simulink model "Square_HFI_Trigger"  (R2022b)
settings: Solver=FixedStepAuto  StartTime=0.0  StopTime=12  FixedStep=1e-7  RelTol=1e-3
undefined symbols (not defined in the file): DiscIntNeverNeededParam, sigbuilder_block
libraries: slpidlib x4, dspsigops x4, dsparch4 x2, simulink x2, spsDCVoltageSourceLib x1, spsPermanentMagnetSynchronousMachineLib x1, dspstat3 x1, spsUniversalBridgeLib x1, spspowerguiLib x1
settings Model: Creator=SSC  LastModifiedBy=SSC

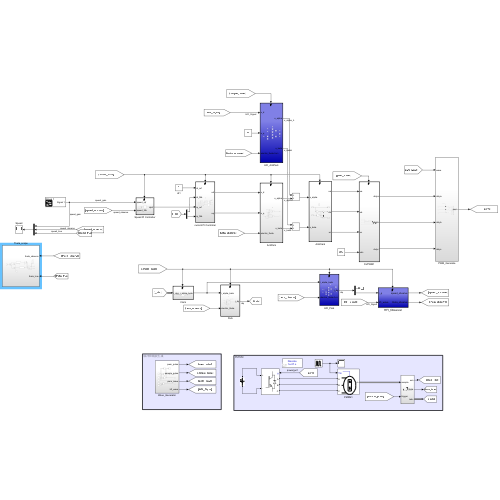
[thumbnail: Simulink's stored preview of the top-level diagram]
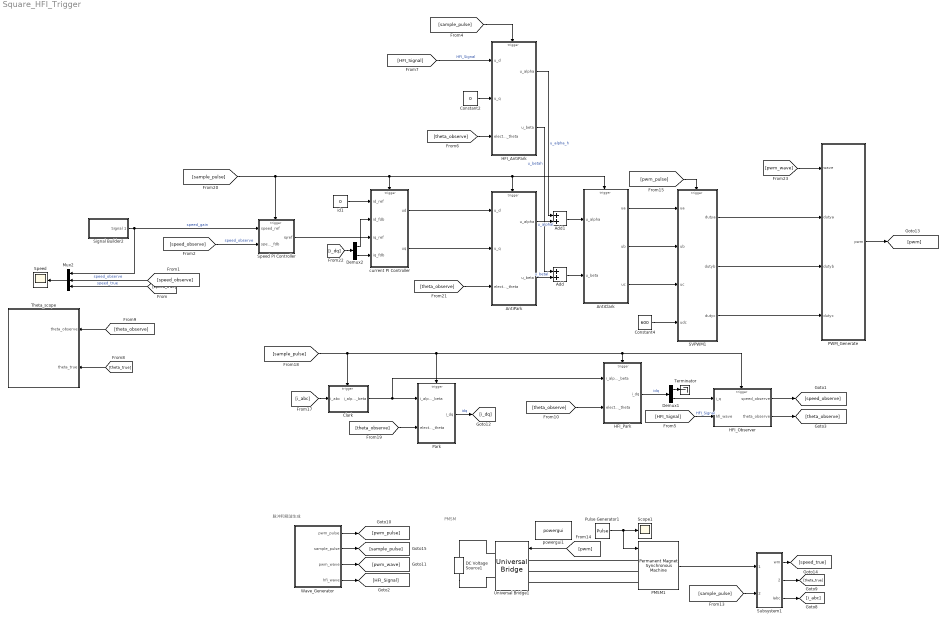
== system Square_HFI_Trigger ==
  note: 脉冲和载波生成
  note: PMSM
  Add : Sum
  Add1 : Sum
  AntiClark : Subsystem
  AntiPark : Subsystem
  Clark : Subsystem
  Constant2 : Constant  Value=0
  Constant4 : Constant  Value=600
  DC Voltage Source1 : spsDCVoltageSourceLib/DC Voltage Source  Amplitude=600  Measurements=None
  Demux1 : Demux  Outputs=2
  Demux2 : Demux  Outputs=2
  HFI_AntiPark : Subsystem
  HFI_Observer : Subsystem
  HFI_Park : Subsystem
  Mux2 : Mux  Inputs=3
  PMSM1 : spsPermanentMagnetSynchronousMachineLib/Permanent Magnet Synchronous Machine  NbPhases=3  FluxDistribution=Sinusoidal  RotorType=Salient-pole  MechanicalLoad=Torque Tm  PresetModel=No  ShowDetailedParameters=on  MeasurementBus=off  Resistance=0.91  Inductance=8.5e-3  dqInductances=[0.00396,0.00796]  La=8.5e-3  MachineConstant=Flux linkage established by magnets (V.s)  Flux=0.446  VoltageCst=161.7909  TorqueCst=1.338  Flat=120  Mechanical=[0.074 0.008 2 0]  PolePairs=4  InitialConditions=[0,0, 0,0]  InitialConditions5ph=[0 0 0 0 0 0]  RefAngle=Aligned with phase A axis (original Park)  IterativeDiscreteModel=Trapezoidal non iterative  TsBlock=-1  TsPowergui=0
  PWM_Generate : Subsystem
  Park : Subsystem
  Pulse Generator1 : DiscretePulseGenerator  PulseType=Time based  Period=3  PulseWidth=33.3  PhaseDelay=2.5
  SVPWM1 : Subsystem
  Scope1 : Scope
  Signal Builder2 : Subsystem  Tag=STV Subsys  LoadFcn=sigbuilder_block('load');  StartFcn=sigbuilder_block('start');  StopFcn=sigbuilder_block('stop');  ClipboardFcn=sigbuilder_block('clipboard');  mask(Sigbuilder block){tuvar=[0:10]}
      mask help: Simulink:masks:SigbuilderBlock_MD
      mask init:
      | if ~strcmp(get_param(bdroot(gcbh),'SimulationStatus'),'stopped') tuvar = sigbuilder_block('maskInit'); end
      settings: CopyFcn=sigbuilder_block('copy');  DeleteFcn=sigbuilder_block('delete');  ModelCloseFcn=sigbuilder_block('modelClose');  PreSaveFcn=sigbuilder_block('preSave');  PauseFcn=sigbuilder_block('pause');  ContinueFcn=sigbuilder_block('continue');  NameChangeFcn=sigbuilder_block('namechange');  OpenFcn=sigbuilder_block('open',[357 166.5 550.5 400.5 ]);  CloseFcn=sigbuilder_block('close');
      mask Display: plot(0, 0, 100, 100,[2, 2, 32, 32, 2], [68, 8, 8, 68, 68],[32, 2], [38, 38], [32, 19, 2],[53, 60, 44], [32, 17, 17, 2],[16, 16, 31, 31]);txt = getActiveGroup(gcbh);text(2, 100, txt,'verticalAlignment', 'top');
  Speed : Scope
  Speed PI Controller : Subsystem  TreatAsAtomicUnit=on
  Subsystem1 : Subsystem
  Terminator : Terminator
  Theta_scope : Subsystem
  Universal Bridge1 : spsUniversalBridgeLib/Universal Bridge  Arms=3  SnubberResistance=1e5  SnubberCapacitance=inf  Device=IGBT / Diodes  Ron=1e-3  Lon=0  ForwardVoltages="[  0  0  ]"  ForwardVoltage=0  GTOparameters=[ 10e-6 , 20e-6 ]  IGBTparameters=[ 1e-6 , 2e-6 ]  Measurements=None  Measurements_2=None  converterType=Rectifier
  Wave_Generator : Subsystem
  current PI Controller : Subsystem
  id1 : Constant  Value=0
  powergui1 : spspowerguiLib/powergui  Priority=1  SimulationMode=Discrete  SampleTime=1e-7  frequency=60  Iterations=50  frequencyindice=0  Pbase=100e6  ErrMax=1e-4  UnitsV=kV  UnitsW=MW  buscounter=0  FunctionMessages=off  echomessages=off  EnableUseOfTLC=off  CurrentSourceSwitches=off  DisableSnubberDevices=off  DisableRonSwitches=off  DisableVfSwitches=off  DisplayEquations=off  AutomaticDiscreteSolvers=off  SolverType=Tustin/Backward Euler (TBE)  Interpol=off  ExternalGateDelay=off  methode=off  Ts=100  x0status=blocks  SPID=on  SwTol=0  HookPort=off  NonlinearTolerance=1e-4  nMaxIteration=100  ContinueOnMaxIteration=off  RestoreLinks=warning  ResistiveCurrentMeasurement=off  Frange=[0:2:500]  Ylog=off  Xlog=on  ShowGrid=off  save=off  variable=ZData  structure=0  ZoomFFT=off  StartTime=0.0  cycles=1  DisplayStyle=1  fundamental=60  FreqAxis=off  MaxFrequency=1000  frequencyindicesteady=1  RmsSteady=1  display=off
  wires:
  Demux1/1 -> Terminator/1
  HFI_Observer/1(speed_observe) -> [speed_observe]
  HFI_Park/1(i_dq) -> Demux1/1  "idq"
  Constant2/1 -> HFI_AntiPark/2(u_q)
  [theta_observe] -> HFI_Park/2(electric_theta)
  [HFI_Signal] -> HFI_AntiPark/1(u_d)  "HFI_Signal"
  [theta_observe] -> HFI_AntiPark/3(electric_theta)
  Mux2/1 -> Speed/1
  [speed_true] -> Mux2/3  "speed_true"
  Demux1/2 -> HFI_Observer/1(i_q)
  [speed_observe] -> Mux2/2  "speed_observe"
  [i_abc] -> Clark/1(i_abc)
  [theta_observe] -> AntiPark/3(electric_theta)
  SVPWM1/3(dutyc) -> PWM_Generate/4(dutyc)
  [theta_observe] -> Park/2(electric_theta)
  current PI Controller/2(uq) -> AntiPark/2(u_q)
  Subsystem1/1(wm) -> [speed_true]
  Wave_Generator/3(pwm_wave) -> [pwm_wave]
  Wave_Generator/2(sample_pulse) -> [sample_pulse]
  [i_dq] -> Demux2/1
  [sample_pulse] -> Speed PI Controller/Trigger, AntiClark/Trigger, AntiPark/Trigger, current PI Controller/Trigger
  Demux2/2 -> current PI Controller/4(iq_fdb)
  Park/1(i_dq) -> [i_dq]  "idq"
  Subsystem1/2(theta) -> [theta_true]
  Speed PI Controller/1(iqref) -> current PI Controller/3(iq_ref)
  SVPWM1/2(dutyb) -> PWM_Generate/3(dutyb)
  Clark/1(i_alpha_beta) -> HFI_Park/1(i_alpha_beta), Park/1(i_alpha_beta)
  Pulse Generator1/1 -> PMSM1/1, Scope1/1
  AntiClark/2(ub) -> SVPWM1/2(ub)
  Signal Builder2/1(Signal 1) -> Mux2/1, Speed PI Controller/1(speed_ref)  "speed_gain"
  PMSM1/1 -> Subsystem1/1(sample)
  Constant4/1 -> SVPWM1/4(udc)
  [pwm_wave] -> PWM_Generate/1(wave)
  [pwm] -> Universal Bridge1/1
  [pwm_pulse] -> SVPWM1/Trigger
  current PI Controller/1(ud) -> AntiPark/1(u_d)
  id1/1 -> current PI Controller/1(id_ref)
  Subsystem1/3(Iabc) -> [i_abc]
  Demux2/1 -> current PI Controller/2(id_fdb)
  PWM_Generate/1(pwm) -> [pwm]
  Wave_Generator/1(pwm_pulse) -> [pwm_pulse]
  [sample_pulse] -> Subsystem1/2(trigger)
  AntiClark/3(uc) -> SVPWM1/3(uc)
  [sample_pulse] -> HFI_Observer/Trigger, HFI_Park/Trigger, Park/Trigger, Clark/Trigger
  SVPWM1/1(dutya) -> PWM_Generate/2(dutya)
  AntiPark/1(u_alpha) -> Add1/2  "u_alphal"
  AntiPark/2(u_beta) -> Add/2  "u_betal"
  Add1/1 -> AntiClark/1(u_alpha)
  AntiClark/1(ua) -> SVPWM1/1(ua)
  Add/1 -> AntiClark/2(u_beta)
  [sample_pulse] -> HFI_AntiPark/Trigger
  Wave_Generator/4(hfi_wave) -> [HFI_Signal]
  [HFI_Signal] -> HFI_Observer/2(hfi_wave)  "HFI_Signal"
  HFI_Observer/2(theta_observe) -> [theta_observe]
  HFI_AntiPark/2(u_beta) -> Add/1  "u_betah"
  HFI_AntiPark/1(u_alpha) -> Add1/1  "u_alpha_h"
  [speed_observe] -> Speed PI Controller/2(speed_fdb)  "speed_observe"
  [theta_observe] -> Theta_scope/1(theta_observe)
  [theta_true] -> Theta_scope/2(theta_true)
  connections:
  PMSM1/LConn1 -- Universal Bridge1/LConn1
  PMSM1/LConn2 -- Universal Bridge1/LConn2
  Universal Bridge1/RConn1 -- DC Voltage Source1/RConn1
  PMSM1/LConn3 -- Universal Bridge1/LConn3
  DC Voltage Source1/LConn1 -- Universal Bridge1/RConn2

== system Square_HFI_Trigger/AntiClark ==
  u_alpha : Inport
  u_beta : Inport  Port=2
  Trigger : TriggerPort  VariantControl=(inherit)
  Gain : Gain  Gain=-1/2
  Gain1 : Gain  Gain=sqrt(3)/2
  Sum : Sum  Inputs=|++
  Sum1 : Sum  Inputs=-+|
  ua : Outport
  ub : Outport  Port=2
  uc : Outport  Port=3
  wires:
  Sum1/1 -> uc/1
  Gain1/1 -> Sum1/1, Sum/2
  Sum/1 -> ub/1
  Gain/1 -> Sum/1, Sum1/2
  u_beta/1 -> Gain1/1
  u_alpha/1 -> ua/1, Gain/1

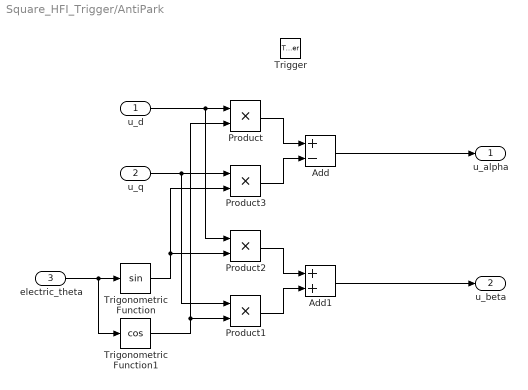
== system Square_HFI_Trigger/AntiPark ==
  u_d : Inport
  u_q : Inport  Port=2
  electric_theta : Inport  Port=3
  Trigger : TriggerPort  VariantControl=(inherit)
  Add : Sum  Inputs=+-
  Add1 : Sum
  Product{,1..3} (4 alike) : Product
  Trigonometric Function : Trigonometry
  Trigonometric Function1 : Trigonometry  Operator=cos
  u_alpha : Outport
  u_beta : Outport  Port=2
  wires:
  electric_theta/1 -> Trigonometric Function1/1, Trigonometric Function/1
  u_d/1 -> Product2/1, Product/1
  Trigonometric Function1/1 -> Product/2, Product1/2
  u_q/1 -> Product1/1, Product3/1
  Trigonometric Function/1 -> Product2/2, Product3/2
  Product/1 -> Add/1
  Product3/1 -> Add/2
  Add/1 -> u_alpha/1
  Product2/1 -> Add1/1
  Product1/1 -> Add1/2
  Add1/1 -> u_beta/1

== system Square_HFI_Trigger/Clark ==
  i_abc : Inport
  Trigger : TriggerPort  VariantControl=(inherit)
  Clark : Subsystem
  Demux : Demux  Outputs=3
  Mux6 : Mux  Inputs=2
  i_alpha_beta : Outport  VectorParamsAs1DForOutWhenUnconnected=off
  wires:
  Clark/2(I_beta) -> Mux6/2
  Mux6/1 -> i_alpha_beta/1
  Demux/3 -> Clark/3(I_c)
  Clark/1(I_alpha) -> Mux6/1
  i_abc/1 -> Demux/1
  Demux/2 -> Clark/2(I_b)
  Demux/1 -> Clark/1(I_a)

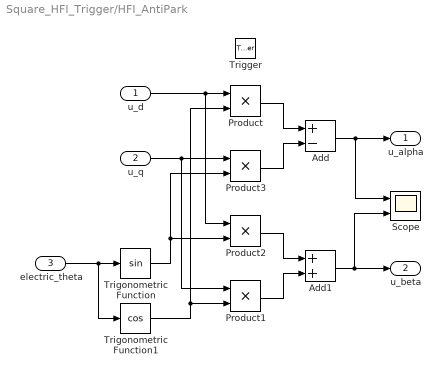
== system Square_HFI_Trigger/HFI_AntiPark ==
  u_d : Inport
  u_q : Inport  Port=2
  electric_theta : Inport  Port=3  LatchByDelayingOutsideSignal=on
  Trigger : TriggerPort  VariantControl=(inherit)
  Add : Sum  Inputs=+-
  Add1 : Sum
  Product{,1..3} (4 alike) : Product
  Scope : Scope  NumInputPorts=2
  Trigonometric Function : Trigonometry
  Trigonometric Function1 : Trigonometry  Operator=cos
  u_alpha : Outport
  u_beta : Outport  Port=2
  wires:
  electric_theta/1 -> Trigonometric Function1/1, Trigonometric Function/1
  u_d/1 -> Product2/1, Product/1
  Trigonometric Function1/1 -> Product/2, Product1/2
  u_q/1 -> Product1/1, Product3/1
  Trigonometric Function/1 -> Product2/2, Product3/2
  Product/1 -> Add/1
  Product3/1 -> Add/2
  Add/1 -> Scope/1, u_alpha/1
  Product2/1 -> Add1/1
  Product1/1 -> Add1/2
  Add1/1 -> Scope/2, u_beta/1

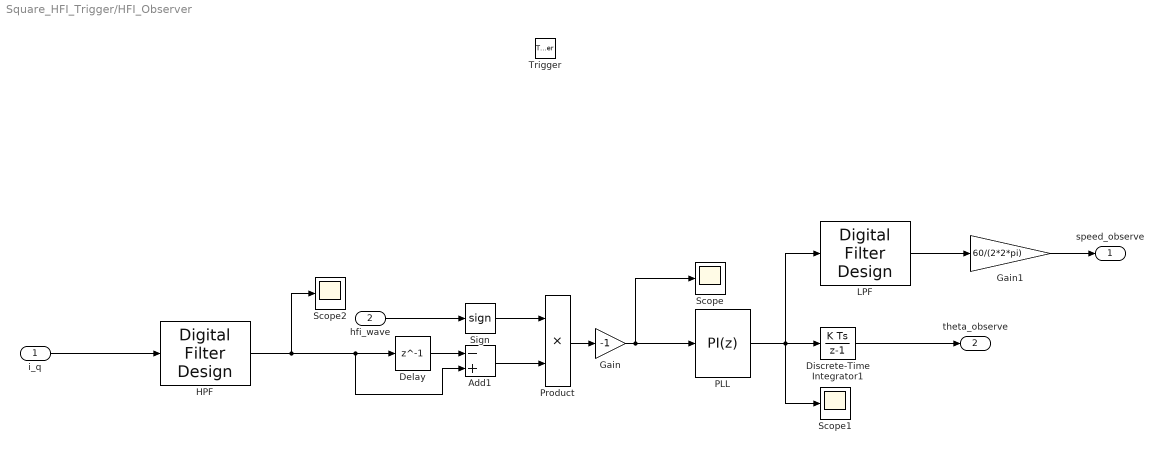
== system Square_HFI_Trigger/HFI_Observer ==
  i_q : Inport
  hfi_wave : Inport  Port=2
  Trigger : TriggerPort  VariantControl=(inherit)
  Add1 : Sum  Inputs=-+
  Delay : Delay  DelayLength=1  InitialCondition=0
  Discrete-Time Integrator1 : DiscreteIntegrator  SampleTime=-1  ICPrevOutput=DiscIntNeverNeededParam  ICPrevScaledInput=DiscIntNeverNeededParam
  Gain : Gain  Gain=-1
  Gain1 : Gain  Gain=60/(2*2*pi)
  HPF : dsparch4/Digital Filter Design  mwdsp_browser_bugfix_var=off
  LPF : dsparch4/Digital Filter Design  mwdsp_browser_bugfix_var=off
  PLL : slpidlib/PID Controller  Controller=PI  Form=Parallel  TimeDomain=Discrete-time  UseExternalTs=off  SampleTime=-1  IntegratorMethod=Forward Euler  FilterMethod=Forward Euler  ControllerParametersSource=internal  P=10000  I=16000/2  UseKiTs=off  D=0  N=100  UseFilter=on  TunerSelectOption=Transfer Function Based (PID Tuner App)  InitialConditionSource=internal  InitialConditionForIntegrator=0  InitialConditionForFilter=0  DifferentiatorICPrevScaledInput=0  ExternalReset=none  TrackingMode=off  Kt=1  LimitOutput=off  SatLimitsSource=internal  UpperSaturationLimit=100*2*pi  LowerSaturationLimit=-100*2*pi  LinearizeAsGain=on  AntiWindupMode=clamping  Kb=1  LimitIntegrator=off  UpperIntegratorSaturationLimit=inf  LowerIntegratorSaturationLimit=-inf  POutMin=[]  POutMax=[]  IOutMin=[]  IOutMax=[]  DOutMin=[]  DOutMax=[]  NOutMin=[]  NOutMax=[]  SumOutMin=[]  SumOutMax=[]  SaturationOutMin=[]  SaturationOutMax=[]  PParamMin=[]  PParamMax=[]  IParamMin=[]  IParamMax=[]  DParamMin=[]  DParamMax=[]  NParamMin=[]  NParamMax=[]  KbParamMin=[]  KbParamMax=[]  KtParamMin=[]  KtParamMax=[]  KbOutMin=[]  KbOutMax=[]  KtOutMin=[]  KtOutMax=[]  IntegratorOutMin=[]  IntegratorOutMax=[]  FilterOutMin=[]  FilterOutMax=[]  SumI1OutMin=[]  SumI1OutMax=[]  SumI2OutMin=[]  SumI2OutMax=[]  SumI3OutMin=[]  SumI3OutMax=[]  SumI4OutMin=[]  SumI4OutMax=[]  SumDOutMin=[]  SumDOutMax=[]  DifferentiatorOutMin=[]  DifferentiatorOutMax=[]  FilterDiffOutCoefMin=[]  FilterDiffOutCoefMax=[]  ReciprocalOutMin=[]  ReciprocalOutMax=[]  SumDenOutMin=[]  SumDenOutMax=[]  SumNumOutMin=[]  SumNumOutMax=[]  DivideOutMin=[]  DivideOutMax=[]  UdiffTsProdOutMin=[]  UdiffTsProdOutMax=[]  NTsProdOutMin=[]  NTsProdOutMax=[]  UintegralTsProdOutMin=[]  UintegralTsProdOutMax=[]  UngainTsProdOutMin=[]  UngainTsProdOutMax=[]  ClampingZeroOutDataTypeStr=Inherit: Inherit via back propagation  ClampingZeroOutMin=[]  ClampingZeroOutMax=[]  FilterDenConstantOutDataTypeStr=Inherit: Inherit via back propagation  FilterDenConstantOutMin=[]  FilterDenConstantOutMax=[]  PCopyOutDataTypeStr=Inherit: Inherit via back propagation  PCopyOutMin=[]  PCopyOutMax=[]  NCopyOutDataTypeStr=Inherit: Inherit via back propagation  NCopyOutMin=[]  NCopyOutMax=[]  IntegratorContinuousStateAttributes=''  IntegratorStateMustResolveToSignalObject=off  IntegratorRTWStateStorageClass=Auto  FilterContinuousStateAttributes=''  FilterStateMustResolveToSignalObject=off  FilterRTWStateStorageClass=Auto  ParallelPVariant=InternalParameters  IdealPVariant=Disabled  IVariant=InternalParameters  DVariant=Disabled  IntegratorVariant=Discrete  SatVariant=Disabled  AWVariant=Passthrough  PCopyVariant=Disabled  TRVariant=Disabled  FdbkBlocksVariant=Forward  IdealPFdbkVariant=Disabled  SatFdbkVariant=Disabled  DerivativeFilterVariant=Disabled  NVariant=Disabled  NCopyVariant=Disabled_SignalSpec  FilterICVariant=Disabled  IntegratorICVariant=InternalICs  ExternalResetVariant=Disabled  TRSumVariant=Passthrough  SumFdbkVariant=Disabled  SumVariant=Sum_PI  TsampFilterVariant=InternalTs  TsampNgainVariant=Passthrough  TsampIntegralVariant=Passthrough  ExternalSaturationOutDataTypeStr=Inherit: Same as second input
  Product : Product
  Scope : Scope
  Scope1 : Scope
  Scope2 : Scope
  Sign : Signum
  speed_observe : Outport  VectorParamsAs1DForOutWhenUnconnected=off
  theta_observe : Outport  Port=2  VectorParamsAs1DForOutWhenUnconnected=off
  wires:
  PLL/1 -> Discrete-Time Integrator1/1, Scope1/1, LPF/1
  Gain1/1 -> speed_observe/1
  LPF/1 -> Gain1/1
  Delay/1 -> Add1/1
  Add1/1 -> Product/2
  Sign/1 -> Product/1
  Product/1 -> Gain/1
  i_q/1 -> HPF/1
  HPF/1 -> Scope2/1, Add1/2, Delay/1
  hfi_wave/1 -> Sign/1
  Discrete-Time Integrator1/1 -> theta_observe/1
  Gain/1 -> Scope/1, PLL/1

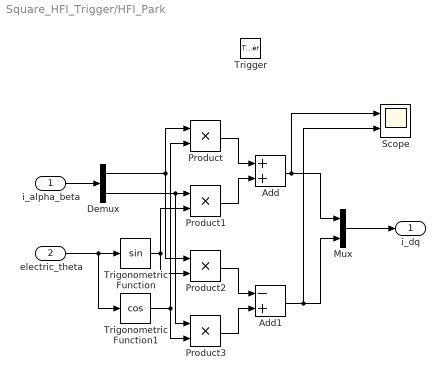
== system Square_HFI_Trigger/HFI_Park ==
  i_alpha_beta : Inport
  electric_theta : Inport  Port=2  LatchByDelayingOutsideSignal=on
  Trigger : TriggerPort  VariantControl=(inherit)
  Add : Sum
  Add1 : Sum  Inputs=-+
  Demux : Demux  Outputs=2
  Mux : Mux  Inputs=2
  Product{,1..3} (4 alike) : Product
  Scope : Scope  NumInputPorts=2
  Trigonometric Function : Trigonometry
  Trigonometric Function1 : Trigonometry  Operator=cos
  i_dq : Outport
  wires:
  electric_theta/1 -> Trigonometric Function1/1, Trigonometric Function/1
  Trigonometric Function1/1 -> Product3/2, Product/2
  Demux/2 -> Product3/1, Product1/1
  Trigonometric Function/1 -> Product2/2, Product1/2
  Product/1 -> Add/1
  Product1/1 -> Add/2
  Product2/1 -> Add1/1
  Product3/1 -> Add1/2
  Add/1 -> Scope/1, Mux/1
  Add1/1 -> Scope/2, Mux/2
  Demux/1 -> Product/1, Product2/1
  i_alpha_beta/1 -> Demux/1
  Mux/1 -> i_dq/1

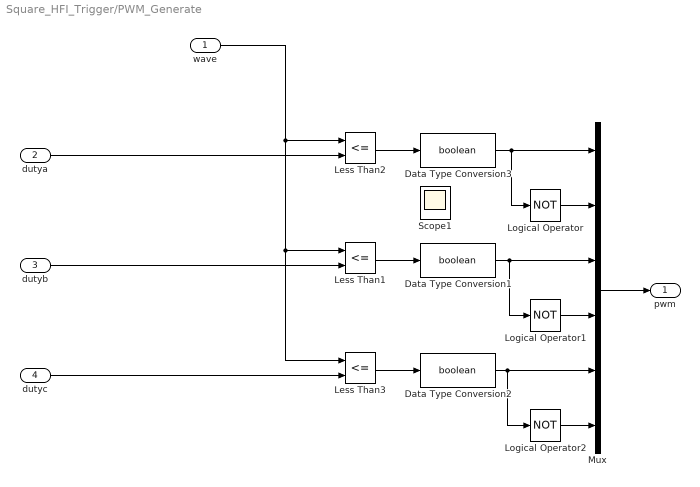
== system Square_HFI_Trigger/PWM_Generate ==
  wave : Inport
  dutya : Inport  Port=2
  dutyb : Inport  Port=3
  dutyc : Inport  Port=4
  Data Type Conversion1 : DataTypeConversion  OutDataTypeStr=boolean  SaturateOnIntegerOverflow=off  RndMeth=Floor
  Data Type Conversion2 : DataTypeConversion  OutDataTypeStr=boolean  SaturateOnIntegerOverflow=off  RndMeth=Floor
  Data Type Conversion3 : DataTypeConversion  OutDataTypeStr=boolean  SaturateOnIntegerOverflow=off  RndMeth=Floor
  Less Than1 : RelationalOperator  Operator=<=  OutDataTypeStr=boolean  RndMeth=Simplest  InputSameDT=off
  Less Than2 : RelationalOperator  Operator=<=  OutDataTypeStr=boolean  RndMeth=Simplest  InputSameDT=off
  Less Than3 : RelationalOperator  Operator=<=  OutDataTypeStr=boolean  RndMeth=Simplest  InputSameDT=off
  Logical Operator : Logic  Operator=NOT  AllPortsSameDT=off  OutDataTypeStr=boolean
  Logical Operator1 : Logic  Operator=NOT  AllPortsSameDT=off  OutDataTypeStr=boolean
  Logical Operator2 : Logic  Operator=NOT  AllPortsSameDT=off  OutDataTypeStr=boolean
  Mux : Mux  Inputs=6
  Scope1 : Scope  NumInputPorts=2
  pwm : Outport
  wires:
  wave/1 -> Less Than3/1, Less Than1/1, Less Than2/1
  Less Than1/1 -> Data Type Conversion1/1
  Less Than2/1 -> Data Type Conversion3/1
  dutyb/1 -> Less Than1/2
  Less Than3/1 -> Data Type Conversion2/1
  dutya/1 -> Less Than2/2
  dutyc/1 -> Less Than3/2
  Data Type Conversion3/1 -> Logical Operator/1, Mux/1
  Logical Operator/1 -> Mux/2
  Data Type Conversion1/1 -> Logical Operator1/1, Mux/3
  Data Type Conversion2/1 -> Logical Operator2/1, Mux/5
  Logical Operator2/1 -> Mux/6
  Mux/1 -> pwm/1
  Logical Operator1/1 -> Mux/4

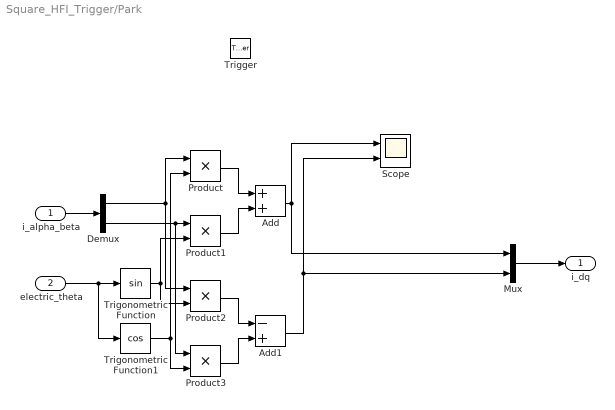
== system Square_HFI_Trigger/Park ==
  i_alpha_beta : Inport
  electric_theta : Inport  Port=2
  Trigger : TriggerPort  VariantControl=(inherit)
  Add : Sum
  Add1 : Sum  Inputs=-+
  Demux : Demux  Outputs=2
  Mux : Mux  Inputs=2
  Product{,1..3} (4 alike) : Product
  Scope : Scope  NumInputPorts=2
  Trigonometric Function : Trigonometry
  Trigonometric Function1 : Trigonometry  Operator=cos
  i_dq : Outport
  wires:
  electric_theta/1 -> Trigonometric Function1/1, Trigonometric Function/1
  Trigonometric Function1/1 -> Product3/2, Product/2
  Demux/2 -> Product3/1, Product1/1
  Trigonometric Function/1 -> Product2/2, Product1/2
  Product/1 -> Add/1
  Product1/1 -> Add/2
  Product2/1 -> Add1/1
  Product3/1 -> Add1/2
  Demux/1 -> Product/1, Product2/1
  i_alpha_beta/1 -> Demux/1
  Mux/1 -> i_dq/1
  Add/1 -> Mux/1, Scope/1
  Add1/1 -> Mux/2, Scope/2

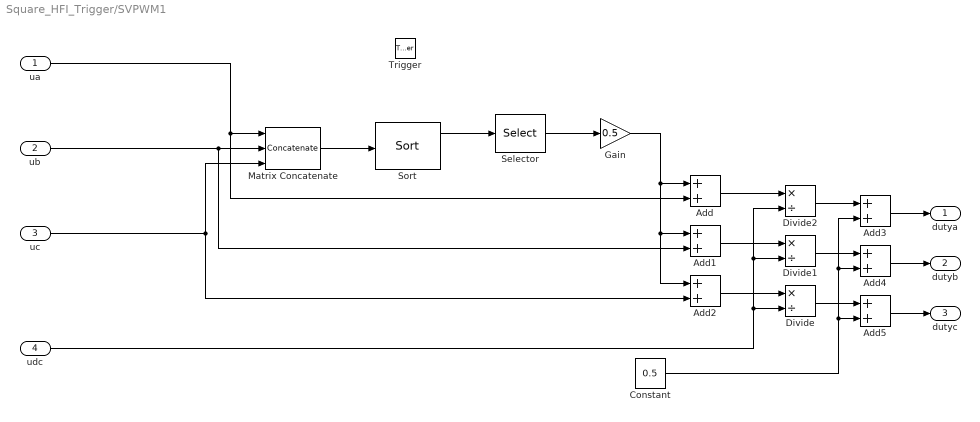
== system Square_HFI_Trigger/SVPWM1 ==
  ua : Inport
  ub : Inport  Port=2
  uc : Inport  Port=3
  udc : Inport  Port=4
  Trigger : TriggerPort  VariantControl=(inherit)
  Add{,1..5} (6 alike) : Sum
  Constant : Constant  Value=0.5
  Divide : Product  Inputs=*/
  Divide1 : Product  Inputs=*/
  Divide2 : Product  Inputs=*/
  Gain : Gain  Gain=0.5
  Matrix Concatenate : Concatenate  NumInputs=3  ConcatenateDimension=2
  Selector : Selector  InputPortWidth=3  IndexOptions=Index vector (dialog)  Indices=2  OutputSizes=1
  Sort : dspstat3/Sort  otype=Value and Index  dir=Ascending  sortAlg=Quick sort  roundingMode=Floor  overflowMode=off  accumDataTypeStr=Inherit: Same as product output  accumLastDataTypeStr=Inherit: Same as product output
  dutya : Outport
  dutyb : Outport  Port=2
  dutyc : Outport  Port=3
  wires:
  Selector/1 -> Gain/1
  udc/1 -> Divide/2, Divide2/2, Divide1/2
  Add1/1 -> Divide1/1
  Sort/1 -> Selector/1
  Matrix Concatenate/1 -> Sort/1
  Add2/1 -> Divide/1
  Gain/1 -> Add2/1, Add1/1, Add/1
  ua/1 -> Add/2, Matrix Concatenate/1
  Add/1 -> Divide2/1
  uc/1 -> Matrix Concatenate/3, Add2/2
  ub/1 -> Add1/2, Matrix Concatenate/2
  Divide2/1 -> Add3/1
  Divide1/1 -> Add4/1
  Divide/1 -> Add5/1
  Constant/1 -> Add5/2, Add4/2, Add3/2
  Add3/1 -> dutya/1
  Add4/1 -> dutyb/1
  Add5/1 -> dutyc/1

== system Square_HFI_Trigger/Signal Builder2 ==
  Demux : Demux  Tag=STV Demux  Outputs=1
      settings: DisplayOption=none
  FromWs : FromWorkspace  Tag=STV FromWs  VariableName=tuvar
      SigBuilderData=|
      | common.afterFinalStr = 'Extrapolate'
      | common.sampleTime = 0
      | dataSet.timeRange = [0 13]
      | dataSet.name = 'Group 1'
      | sbobj.Groups.Name = 'Group 1'
      | sbobj.Groups.Signals.Name = 'Signal 1'
      | sbobj.Groups.Signals.XData = [0 0.5 0.51 8 8 13]
      | sbobj.Groups.Signals.YData = [0 0 50 50 40 40]
      | sbobj.Groups.TimeRange = [0 13]
  Signal 1 : Outport  Tag=STV Outport
  wires:
  FromWs/1 -> Demux/1
  Demux/1 -> Signal 1/1

== system Square_HFI_Trigger/Speed PI Controller ==
  speed_ref : Inport
  speed_fdb : Inport  Port=2
  Trigger : TriggerPort  VariantControl=(inherit)
  Speed PI Controller : slpidlib/PID Controller  Controller=PI  Form=Parallel  TimeDomain=Discrete-time  UseExternalTs=off  SampleTime=-1  IntegratorMethod=Forward Euler  FilterMethod=Forward Euler  ControllerParametersSource=internal  P=3.786/30  I=44.84/30/2  UseKiTs=off  D=0  N=100  UseFilter=on  TunerSelectOption=Transfer Function Based (PID Tuner App)  InitialConditionSource=internal  InitialConditionForIntegrator=0  InitialConditionForFilter=0  DifferentiatorICPrevScaledInput=0  ExternalReset=none  TrackingMode=off  Kt=1  LimitOutput=off  SatLimitsSource=internal  UpperSaturationLimit=5.65  LowerSaturationLimit=-5.65  LinearizeAsGain=on  AntiWindupMode=clamping  Kb=1  LimitIntegrator=off  UpperIntegratorSaturationLimit=inf  LowerIntegratorSaturationLimit=-inf  POutMin=[]  POutMax=[]  IOutMin=[]  IOutMax=[]  DOutMin=[]  DOutMax=[]  NOutMin=[]  NOutMax=[]  SumOutMin=[]  SumOutMax=[]  SaturationOutMin=[]  SaturationOutMax=[]  PParamMin=[]  PParamMax=[]  IParamMin=[]  IParamMax=[]  DParamMin=[]  DParamMax=[]  NParamMin=[]  NParamMax=[]  KbParamMin=[]  KbParamMax=[]  KtParamMin=[]  KtParamMax=[]  KbOutMin=[]  KbOutMax=[]  KtOutMin=[]  KtOutMax=[]  IntegratorOutMin=[]  IntegratorOutMax=[]  FilterOutMin=[]  FilterOutMax=[]  SumI1OutMin=[]  SumI1OutMax=[]  SumI2OutMin=[]  SumI2OutMax=[]  SumI3OutMin=[]  SumI3OutMax=[]  SumI4OutMin=[]  SumI4OutMax=[]  SumDOutMin=[]  SumDOutMax=[]  DifferentiatorOutMin=[]  DifferentiatorOutMax=[]  FilterDiffOutCoefMin=[]  FilterDiffOutCoefMax=[]  ReciprocalOutMin=[]  ReciprocalOutMax=[]  SumDenOutMin=[]  SumDenOutMax=[]  SumNumOutMin=[]  SumNumOutMax=[]  DivideOutMin=[]  DivideOutMax=[]  UdiffTsProdOutMin=[]  UdiffTsProdOutMax=[]  NTsProdOutMin=[]  NTsProdOutMax=[]  UintegralTsProdOutMin=[]  UintegralTsProdOutMax=[]  UngainTsProdOutMin=[]  UngainTsProdOutMax=[]  ClampingZeroOutDataTypeStr=Inherit: Inherit via back propagation  ClampingZeroOutMin=[]  ClampingZeroOutMax=[]  FilterDenConstantOutDataTypeStr=Inherit: Inherit via back propagation  FilterDenConstantOutMin=[]  FilterDenConstantOutMax=[]  PCopyOutDataTypeStr=Inherit: Inherit via back propagation  PCopyOutMin=[]  PCopyOutMax=[]  NCopyOutDataTypeStr=Inherit: Inherit via back propagation  NCopyOutMin=[]  NCopyOutMax=[]  IntegratorContinuousStateAttributes=''  IntegratorStateMustResolveToSignalObject=off  IntegratorRTWStateStorageClass=Auto  FilterContinuousStateAttributes=''  FilterStateMustResolveToSignalObject=off  FilterRTWStateStorageClass=Auto  ParallelPVariant=InternalParameters  IdealPVariant=Disabled  IVariant=InternalParameters  DVariant=Disabled  IntegratorVariant=Discrete  SatVariant=Disabled  AWVariant=Passthrough  PCopyVariant=Disabled  TRVariant=Disabled  FdbkBlocksVariant=Forward  IdealPFdbkVariant=Disabled  SatFdbkVariant=Disabled  DerivativeFilterVariant=Disabled  NVariant=Disabled  NCopyVariant=Disabled_SignalSpec  FilterICVariant=Disabled  IntegratorICVariant=InternalICs  ExternalResetVariant=Disabled  TRSumVariant=Passthrough  SumFdbkVariant=Disabled  SumVariant=Sum_PI  TsampFilterVariant=InternalTs  TsampNgainVariant=Passthrough  TsampIntegralVariant=Passthrough  ExternalSaturationOutDataTypeStr=Inherit: Same as second input
  Sum3 : Sum  Inputs=|+-
  iqref : Outport
  wires:
  Sum3/1 -> Speed PI Controller/1
  Speed PI Controller/1 -> iqref/1
  speed_ref/1 -> Sum3/1
  speed_fdb/1 -> Sum3/2

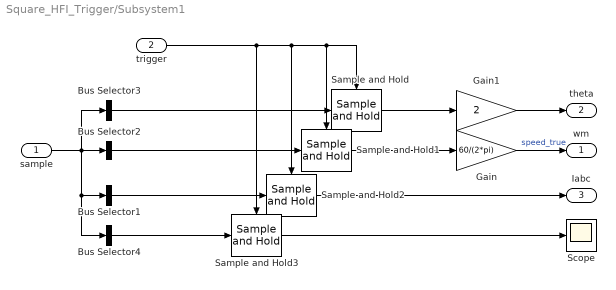
== system Square_HFI_Trigger/Subsystem1 ==
  sample : Inport
  trigger : Inport  Port=2
  Bus Selector1 : BusSelector  OutputSignals=Stator current is_a (A),Stator current is_b (A),Stator current is_c (A)  OutputAsBus=on
  Bus Selector2 : BusSelector  OutputSignals=Rotor speed wm (rad/s)  OutputAsBus=on
  Bus Selector3 : BusSelector  OutputSignals=Rotor angle thetam (rad)  OutputAsBus=on
  Bus Selector4 : BusSelector  OutputSignals=Rotor speed wm (rad/s)  OutputAsBus=on
  Gain : Gain  Gain=60/(2*pi)
  Gain1 : Gain  Gain=2
  Sample and Hold{,1..3} (4 alike) : dspsigops/Sample and Hold  trig=Rising edge  initCond=0  latchinput=off
  Scope : Scope
  wm : Outport  VectorParamsAs1DForOutWhenUnconnected=off
  theta : Outport  Port=2  VectorParamsAs1DForOutWhenUnconnected=off
  Iabc : Outport  Port=3  VectorParamsAs1DForOutWhenUnconnected=off
  wires:
  sample/1 -> Bus Selector4/1, Bus Selector1/1, Bus Selector3/1, Bus Selector2/1
  Gain/1 -> wm/1  "speed_true"
  Gain1/1 -> theta/1
  Sample and Hold/1 -> Gain1/1
  Bus Selector3/1 -> Sample and Hold/1
  Sample and Hold1/1 -> Gain/1
  Bus Selector2/1 -> Sample and Hold1/1
  Bus Selector1/1 -> Sample and Hold2/1
  Sample and Hold2/1 -> Iabc/1
  Bus Selector4/1 -> Sample and Hold3/1
  Sample and Hold3/1 -> Scope/1
  trigger/1 -> Sample and Hold3/Trigger, Sample and Hold2/Trigger, Sample and Hold1/Trigger, Sample and Hold/Trigger

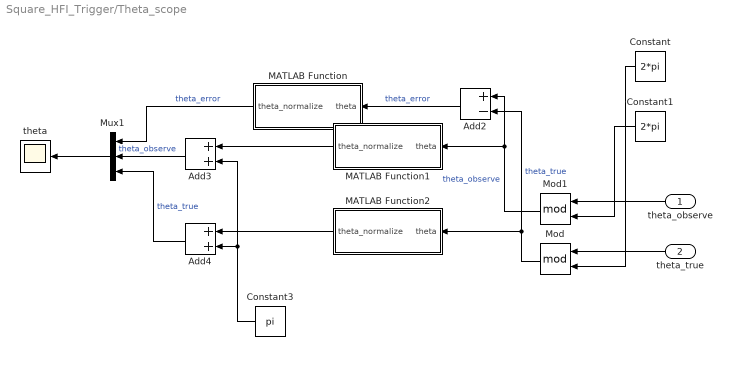
== system Square_HFI_Trigger/Theta_scope ==
  theta_observe : Inport
  theta_true : Inport  Port=2
  Add2 : Sum  Inputs=+-
  Add3 : Sum
  Add4 : Sum
  Constant : Constant  Value=2*pi
  Constant1 : Constant  Value=2*pi
  Constant3 : Constant  Value=pi
  MATLAB Function : MATLAB Function  TreatAsAtomicUnit=on
  MATLAB Function1 : MATLAB Function  TreatAsAtomicUnit=on
  MATLAB Function2 : MATLAB Function  TreatAsAtomicUnit=on
  Mod : Math  Operator=mod  SignedPower=on
  Mod1 : Math  Operator=mod  SignedPower=on
  Mux1 : Mux  Inputs=3
  theta : Scope
  wires:
  Add4/1 -> Mux1/3  "theta_true"
  Constant1/1 -> Mod1/2
  Constant/1 -> Mod/2
  MATLAB Function2/1(theta_normalize) -> Add4/1
  Mod/1 -> Add2/2, MATLAB Function2/1(theta)  "theta_true"
  Mux1/1 -> theta/1
  theta_observe/1 -> Mod1/1
  Constant3/1 -> Add4/2, Add3/2
  MATLAB Function/1(theta_normalize) -> Mux1/1  "theta_error"
  MATLAB Function1/1(theta_normalize) -> Add3/1
  Mod1/1 -> Add2/1, MATLAB Function1/1(theta)  "theta_observe"
  Add3/1 -> Mux1/2  "theta_observe"
  Add2/1 -> MATLAB Function/1(theta)  "theta_error"
  theta_true/1 -> Mod/1

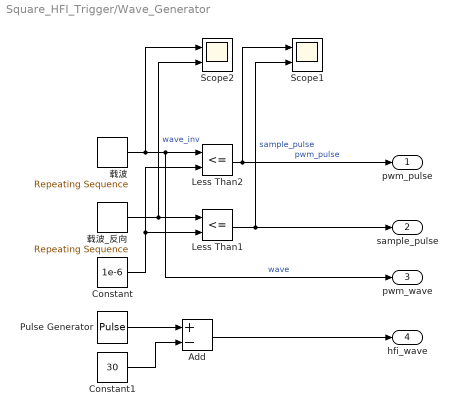
== system Square_HFI_Trigger/Wave_Generator ==
  Add : Sum  Inputs=+-
  Constant : Constant  Value=1e-6
  Constant1 : Constant  Value=30
  Less Than1 : RelationalOperator  Operator=<=  OutDataTypeStr=boolean  RndMeth=Simplest  InputSameDT=off
  Less Than2 : RelationalOperator  Operator=<=  OutDataTypeStr=boolean  RndMeth=Simplest  InputSameDT=off
  Pulse Generator : DiscretePulseGenerator  PulseType=Time based  Amplitude=60  Period=2e-4  PulseWidth=50
  Scope1 : Scope  NumInputPorts=2
  Scope2 : Scope  NumInputPorts=2
  载波 : simulink/Sources/Repeating Sequence  rep_seq_t=[0 0.5e-4 1e-4]  rep_seq_y=[0 1 0]
  载波_反向 : simulink/Sources/Repeating Sequence  rep_seq_t=[0 0.5e-4 1e-4]  rep_seq_y=[1 0 1]
  pwm_pulse : Outport
  sample_pulse : Outport  Port=2
  pwm_wave : Outport  Port=3
  hfi_wave : Outport  Port=4
  wires:
  Less Than2/1 -> pwm_pulse/1, Scope1/1  "pwm_pulse"
  Constant/1 -> Less Than1/2, Less Than2/2
  载波/1 -> pwm_wave/1, Less Than2/1, Scope2/1  "wave"
  Less Than1/1 -> sample_pulse/1, Scope1/2  "sample_pulse"
  载波_反向/1 -> Scope2/2, Less Than1/1  "wave_inv"
  Pulse Generator/1 -> Add/1
  Add/1 -> hfi_wave/1
  Constant1/1 -> Add/2

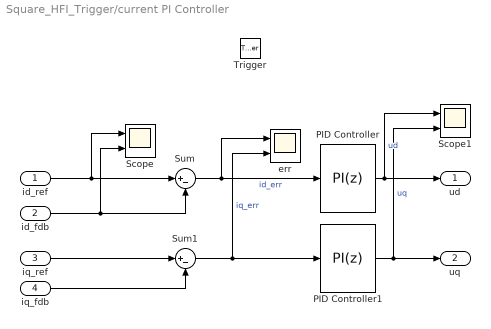
== system Square_HFI_Trigger/current PI Controller ==
  id_ref : Inport
  id_fdb : Inport  Port=2
  iq_ref : Inport  Port=3
  iq_fdb : Inport  Port=4
  Trigger : TriggerPort  VariantControl=(inherit)
  PID Controller : slpidlib/PID Controller  Controller=PI  Form=Parallel  TimeDomain=Discrete-time  UseExternalTs=off  SampleTime=-1  IntegratorMethod=Forward Euler  FilterMethod=Forward Euler  ControllerParametersSource=internal  P=19.8  I=4550  UseKiTs=off  D=0  N=100  UseFilter=on  TunerSelectOption=Transfer Function Based (PID Tuner App)  InitialConditionSource=internal  InitialConditionForIntegrator=0  InitialConditionForFilter=0  DifferentiatorICPrevScaledInput=0  ExternalReset=none  TrackingMode=off  Kt=1  LimitOutput=on  SatLimitsSource=internal  UpperSaturationLimit=600/sqrt(3)  LowerSaturationLimit=-600/sqrt(3)  LinearizeAsGain=on  AntiWindupMode=clamping  Kb=1  LimitIntegrator=off  UpperIntegratorSaturationLimit=inf  LowerIntegratorSaturationLimit=-inf  POutMin=[]  POutMax=[]  IOutMin=[]  IOutMax=[]  DOutMin=[]  DOutMax=[]  NOutMin=[]  NOutMax=[]  SumOutMin=[]  SumOutMax=[]  SaturationOutMin=[]  SaturationOutMax=[]  PParamMin=[]  PParamMax=[]  IParamMin=[]  IParamMax=[]  DParamMin=[]  DParamMax=[]  NParamMin=[]  NParamMax=[]  KbParamMin=[]  KbParamMax=[]  KtParamMin=[]  KtParamMax=[]  KbOutMin=[]  KbOutMax=[]  KtOutMin=[]  KtOutMax=[]  IntegratorOutMin=[]  IntegratorOutMax=[]  FilterOutMin=[]  FilterOutMax=[]  SumI1OutMin=[]  SumI1OutMax=[]  SumI2OutMin=[]  SumI2OutMax=[]  SumI3OutMin=[]  SumI3OutMax=[]  SumI4OutMin=[]  SumI4OutMax=[]  SumDOutMin=[]  SumDOutMax=[]  DifferentiatorOutMin=[]  DifferentiatorOutMax=[]  FilterDiffOutCoefMin=[]  FilterDiffOutCoefMax=[]  ReciprocalOutMin=[]  ReciprocalOutMax=[]  SumDenOutMin=[]  SumDenOutMax=[]  SumNumOutMin=[]  SumNumOutMax=[]  DivideOutMin=[]  DivideOutMax=[]  UdiffTsProdOutMin=[]  UdiffTsProdOutMax=[]  NTsProdOutMin=[]  NTsProdOutMax=[]  UintegralTsProdOutMin=[]  UintegralTsProdOutMax=[]  UngainTsProdOutMin=[]  UngainTsProdOutMax=[]  ClampingZeroOutDataTypeStr=Inherit: Inherit via back propagation  ClampingZeroOutMin=[]  ClampingZeroOutMax=[]  FilterDenConstantOutDataTypeStr=Inherit: Inherit via back propagation  FilterDenConstantOutMin=[]  FilterDenConstantOutMax=[]  PCopyOutDataTypeStr=Inherit: Inherit via back propagation  PCopyOutMin=[]  PCopyOutMax=[]  NCopyOutDataTypeStr=Inherit: Inherit via back propagation  NCopyOutMin=[]  NCopyOutMax=[]  IntegratorContinuousStateAttributes=''  IntegratorStateMustResolveToSignalObject=off  IntegratorRTWStateStorageClass=Auto  FilterContinuousStateAttributes=''  FilterStateMustResolveToSignalObject=off  FilterRTWStateStorageClass=Auto  ParallelPVariant=InternalParameters  IdealPVariant=Disabled  IVariant=InternalParameters  DVariant=Disabled  IntegratorVariant=Discrete  SatVariant=Enabled  AWVariant=DiscClampingParallel  PCopyVariant=Disabled  TRVariant=Disabled  FdbkBlocksVariant=Forward  IdealPFdbkVariant=Disabled  SatFdbkVariant=Disabled  DerivativeFilterVariant=Disabled  NVariant=Disabled  NCopyVariant=Disabled_SignalSpec  FilterICVariant=Disabled  IntegratorICVariant=InternalICs  ExternalResetVariant=Disabled  TRSumVariant=Passthrough  SumFdbkVariant=Disabled  SumVariant=Sum_PI  TsampFilterVariant=InternalTs  TsampNgainVariant=Passthrough  TsampIntegralVariant=Passthrough  ExternalSaturationOutDataTypeStr=Inherit: Same as second input
  PID Controller1 : slpidlib/PID Controller  Controller=PI  Form=Parallel  TimeDomain=Discrete-time  UseExternalTs=off  SampleTime=-1  IntegratorMethod=Forward Euler  FilterMethod=Forward Euler  ControllerParametersSource=internal  P=19.8  I=4550  UseKiTs=off  D=0  N=100  UseFilter=on  TunerSelectOption=Transfer Function Based (PID Tuner App)  InitialConditionSource=internal  InitialConditionForIntegrator=0  InitialConditionForFilter=0  DifferentiatorICPrevScaledInput=0  ExternalReset=none  TrackingMode=off  Kt=1  LimitOutput=on  SatLimitsSource=internal  UpperSaturationLimit=600/sqrt(3)  LowerSaturationLimit=-600/sqrt(3)  LinearizeAsGain=on  AntiWindupMode=clamping  Kb=1  LimitIntegrator=off  UpperIntegratorSaturationLimit=inf  LowerIntegratorSaturationLimit=-inf  POutMin=[]  POutMax=[]  IOutMin=[]  IOutMax=[]  DOutMin=[]  DOutMax=[]  NOutMin=[]  NOutMax=[]  SumOutMin=[]  SumOutMax=[]  SaturationOutMin=[]  SaturationOutMax=[]  PParamMin=[]  PParamMax=[]  IParamMin=[]  IParamMax=[]  DParamMin=[]  DParamMax=[]  NParamMin=[]  NParamMax=[]  KbParamMin=[]  KbParamMax=[]  KtParamMin=[]  KtParamMax=[]  KbOutMin=[]  KbOutMax=[]  KtOutMin=[]  KtOutMax=[]  IntegratorOutMin=[]  IntegratorOutMax=[]  FilterOutMin=[]  FilterOutMax=[]  SumI1OutMin=[]  SumI1OutMax=[]  SumI2OutMin=[]  SumI2OutMax=[]  SumI3OutMin=[]  SumI3OutMax=[]  SumI4OutMin=[]  SumI4OutMax=[]  SumDOutMin=[]  SumDOutMax=[]  DifferentiatorOutMin=[]  DifferentiatorOutMax=[]  FilterDiffOutCoefMin=[]  FilterDiffOutCoefMax=[]  ReciprocalOutMin=[]  ReciprocalOutMax=[]  SumDenOutMin=[]  SumDenOutMax=[]  SumNumOutMin=[]  SumNumOutMax=[]  DivideOutMin=[]  DivideOutMax=[]  UdiffTsProdOutMin=[]  UdiffTsProdOutMax=[]  NTsProdOutMin=[]  NTsProdOutMax=[]  UintegralTsProdOutMin=[]  UintegralTsProdOutMax=[]  UngainTsProdOutMin=[]  UngainTsProdOutMax=[]  ClampingZeroOutDataTypeStr=Inherit: Inherit via back propagation  ClampingZeroOutMin=[]  ClampingZeroOutMax=[]  FilterDenConstantOutDataTypeStr=Inherit: Inherit via back propagation  FilterDenConstantOutMin=[]  FilterDenConstantOutMax=[]  PCopyOutDataTypeStr=Inherit: Inherit via back propagation  PCopyOutMin=[]  PCopyOutMax=[]  NCopyOutDataTypeStr=Inherit: Inherit via back propagation  NCopyOutMin=[]  NCopyOutMax=[]  IntegratorContinuousStateAttributes=''  IntegratorStateMustResolveToSignalObject=off  IntegratorRTWStateStorageClass=Auto  FilterContinuousStateAttributes=''  FilterStateMustResolveToSignalObject=off  FilterRTWStateStorageClass=Auto  ParallelPVariant=InternalParameters  IdealPVariant=Disabled  IVariant=InternalParameters  DVariant=Disabled  IntegratorVariant=Discrete  SatVariant=Enabled  AWVariant=DiscClampingParallel  PCopyVariant=Disabled  TRVariant=Disabled  FdbkBlocksVariant=Forward  IdealPFdbkVariant=Disabled  SatFdbkVariant=Disabled  DerivativeFilterVariant=Disabled  NVariant=Disabled  NCopyVariant=Disabled_SignalSpec  FilterICVariant=Disabled  IntegratorICVariant=InternalICs  ExternalResetVariant=Disabled  TRSumVariant=Passthrough  SumFdbkVariant=Disabled  SumVariant=Sum_PI  TsampFilterVariant=InternalTs  TsampNgainVariant=Passthrough  TsampIntegralVariant=Passthrough  ExternalSaturationOutDataTypeStr=Inherit: Same as second input
  Scope : Scope  NumInputPorts=2
  Scope1 : Scope  NumInputPorts=2
  Sum : Sum  Inputs=|+-
  Sum1 : Sum  Inputs=|+-
  err : Scope  NumInputPorts=2
  ud : Outport
  uq : Outport  Port=2
  wires:
  iq_fdb/1 -> Sum1/2
  Sum1/1 -> PID Controller1/1, err/2  "iq_err"
  id_fdb/1 -> Scope/2, Sum/2
  Sum/1 -> err/1, PID Controller/1  "id_err"
  id_ref/1 -> Scope/1, Sum/1
  iq_ref/1 -> Sum1/1
  PID Controller1/1 -> Scope1/2, uq/1  "uq"
  PID Controller/1 -> Scope1/1, ud/1  "ud"

== system Square_HFI_Trigger/Clark/Clark ==
  I_a : Inport
  I_b : Inport  Port=2
  I_c : Inport  Port=3
  Add : Sum
  Add1 : Sum  Inputs=+-
  Add2 : Sum  Inputs=+-
  Gain : Gain  Gain=2/3
  Gain1 : Gain  Gain=1/3
  Gain2 : Gain  Gain=sqrt(3)/3
  I_alpha : Outport
  I_beta : Outport  Port=2
  wires:
  I_a/1 -> Gain/1
  I_b/1 -> Add1/1, Add/1
  I_c/1 -> Add/2, Add1/2
  Add/1 -> Gain1/1
  Add1/1 -> Gain2/1
  Gain/1 -> Add2/1
  Gain1/1 -> Add2/2
  Add2/1 -> I_alpha/1
  Gain2/1 -> I_beta/1

== matlab function Square_HFI_Trigger/Theta_scope/MATLAB Function ==
  data: theta input; theta_normalize output
function theta_normalize = fcn(theta)
if (theta > pi)
    theta = theta - 2 * pi;
elseif (theta< -pi)
    theta = theta + 2 * pi;
end
theta_normalize = theta;

== matlab function Square_HFI_Trigger/Theta_scope/MATLAB Function2 ==
  data: theta input; theta_normalize output
function theta_normalize = fcn(theta)
if (theta > pi)
    theta = theta - 2 * pi;
elseif (theta< -pi)
    theta = theta + 2 * pi;
end
theta_normalize = theta;

== matlab function Square_HFI_Trigger/Theta_scope/MATLAB Function1 ==
  data: theta input; theta_normalize output
function theta_normalize = fcn(theta)
if (theta > pi)
    theta = theta - 2 * pi;
elseif (theta< -pi)
    theta = theta + 2 * pi;
end
theta_normalize = theta;
